simulink model "esercitazione3"  (R2023b)
settings: Solver=VariableStepAuto  StartTime=0.0  StopTime=12000  MaxStep=0.01  RelTol=1e-3
InitFcn:
  | init3
values from neighbouring files (symbols this model uses):
  B = 1.02e-9/60    (= 1.7e-11)    [init3.m]
  cp = 2*eps*sqrt(kp*mp)    [init3.m]
  d_sp = [0.001; 0.003; 0.005]    [init3.m]
  I = [I_x; I_y; I_z]    [init3.m]
  i = 0    [init3.m]
  Iw = Hm/wmax    (= 2.02922552442e-06)    [init3.m]
  Km = 1.09e-3    (= 0.00109)    [init3.m]
  kp = kt/(Lp^2)    (= 0.05)    [init3.m]
  Kprp = Km*Kv/Iw*20    (= 11.7098862172)    [init3.m]
  Kv = Km    (= 0.00109)    [init3.m]
  Lp = 0.2    [init3.m]
  mp = 0.146    [init3.m]
  mu = 398600    [init3.m]
  q_0 = [1; 0; 0; 0]    [init3.m]
  r_o = h+R_E    (= 7095.14)    [init3.m]
  Rm = 8.8    [init3.m]
  w_ic = [0; -w_o; 0]    [init3.m]
  w_o = sqrt(mu/(h+R_E)^3)    [init3.m]
  y_0 = [0; -w_o; 0; 0; 0]    [init3.m]
undefined symbols (not defined in the file or in its folder): C_phi, C_psi, C_theta
libraries: simulink x4, matrix_library x1
settings Model: Creator=dario  LastModifiedBy=Francesco

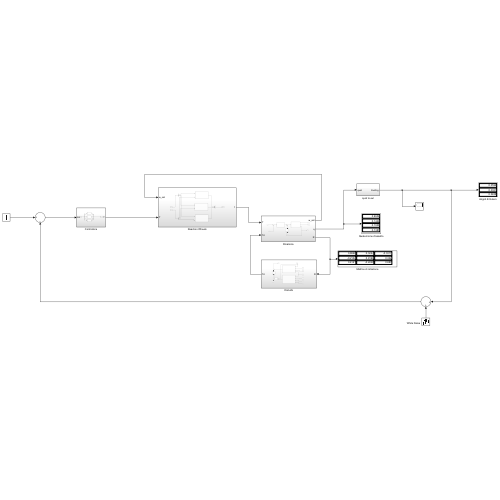
[thumbnail: Simulink's stored preview of the top-level diagram]
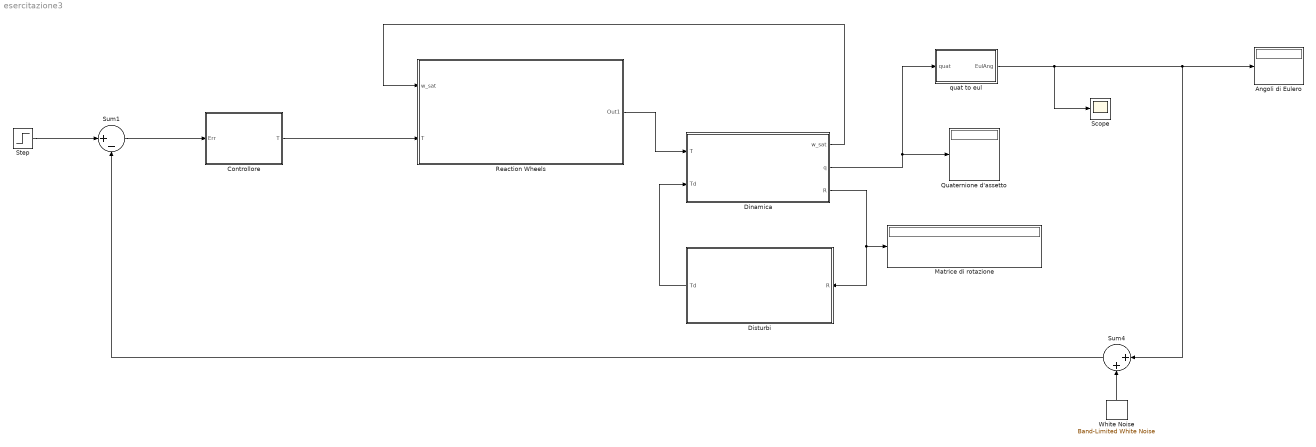
== system esercitazione3 ==
  " White Noise" : simulink/Sources/Band-Limited White Noise  Cov=[1e-6]  Ts=0.1  seed=[23341]
  Angoli di Eulero : Display
  Controllore : Subsystem
  Dinamica : Subsystem
  Disturbi : Subsystem
  Matrice di rotazione : Display
  Quaternione d'assetto : Display
  Reaction Wheels : Subsystem
  Scope : Scope
  Step : Step  After=20*pi/180  SampleTime=0  VectorParams1D=off
  Sum1 : Sum  Inputs=|+-
  Sum4 : Sum  Inputs=|++
  quat to eul : Subsystem
  wires:
  quat to eul/1(EulAng) -> Sum4/1, Angoli di Eulero/1, Scope/1
  Step/1 -> Sum1/1
  Sum1/1 -> Controllore/1(Err)
  Dinamica/2(q) -> quat to eul/1(quat), Quaternione d'assetto/1
  Controllore/1(T) -> Reaction Wheels/2(T)
  Dinamica/3(R) -> Disturbi/1(R), Matrice di rotazione/1
  Disturbi/1(Td) -> Dinamica/2(Td)
  " White Noise"/1 -> Sum4/2
  Sum4/1 -> Sum1/2
  Reaction Wheels/1(Out1) -> Dinamica/1(T)
  Dinamica/1(w_sat) -> Reaction Wheels/1(w_sat)

== system esercitazione3/Controllore ==
  Err : Inport
  C_phi : ZeroPole  Zeros=-0.00107058950149057  Poles=-1.61866208436204  Gain=C_phi.K
  C_psi : ZeroPole  Zeros=-0.000407767798417688  Poles=-1.39195940880825  Gain=C_psi.K
  C_th : ZeroPole  Zeros=-0.000686475078764194  Poles=-0.555984695028282  Gain=C_theta.K
  Demux : Demux  Outputs=3
  Mux : Mux  Inputs=3
  T : Outport
  wires:
  Demux/1 -> C_phi/1
  C_th/1 -> Mux/2
  C_psi/1 -> Mux/3
  Demux/3 -> C_psi/1
  Err/1 -> Demux/1
  Demux/2 -> C_th/1
  C_phi/1 -> Mux/1
  Mux/1 -> T/1

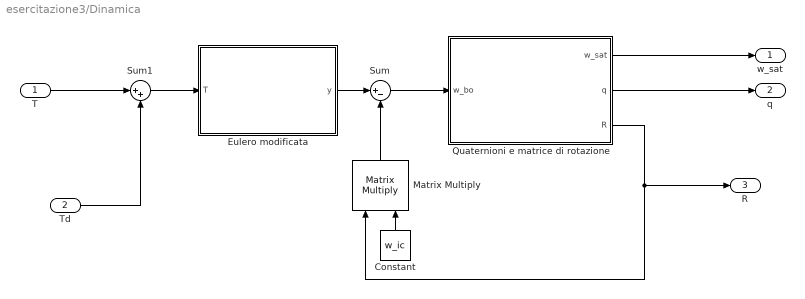
== system esercitazione3/Dinamica ==
  T : Inport
  Td : Inport  Port=2
  Constant : Constant  Value=w_ic  VectorParams1D=off
  "Eulero modificata " : Subsystem
  Matrix Multiply : Product  Inputs=**  Multiplication=Matrix(*)
  Quaternioni e matrice di rotazione : Subsystem
  Sum : Sum  Inputs=|+-
  Sum1 : Sum  Inputs=|++
  w_sat : Outport
  q : Outport  Port=2
  R : Outport  Port=3
  wires:
  Sum/1 -> Quaternioni e matrice di rotazione/1(w_bo)
  Constant/1 -> Matrix Multiply/2
  Quaternioni e matrice di rotazione/2(q) -> q/1
  Quaternioni e matrice di rotazione/3(R) -> R/1, Matrix Multiply/1
  Matrix Multiply/1 -> Sum/2
  T/1 -> Sum1/1
  Td/1 -> Sum1/2
  Sum1/1 -> "Eulero modificata "/1(T)
  "Eulero modificata "/1(y) -> Sum/1
  Quaternioni e matrice di rotazione/1(w_sat) -> w_sat/1

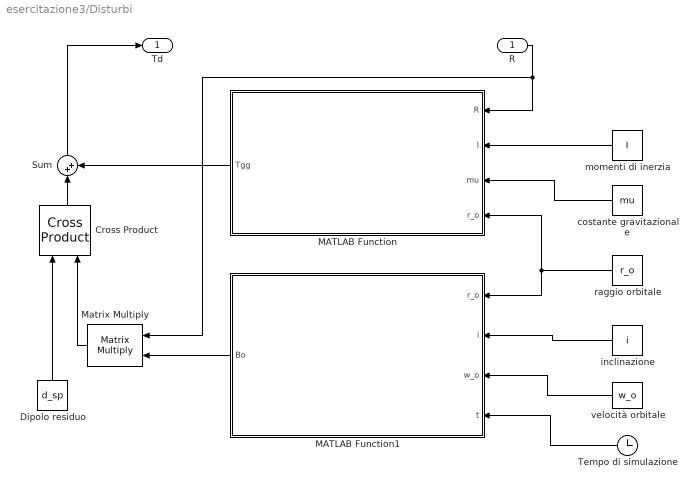
== system esercitazione3/Disturbi ==
  R : Inport
  Cross Product : matrix_library/Cross Product
  Dipolo residuo : Constant  Value=d_sp  VectorParams1D=off
  MATLAB Function : MATLAB Function  TreatAsAtomicUnit=on
  MATLAB Function1 : MATLAB Function  TreatAsAtomicUnit=on
  Matrix Multiply : Product  Inputs=**  Multiplication=Matrix(*)
  Sum : Sum  Inputs=|++
  Tempo di simulazione : Clock
  costante gravitazionale : Constant  Value=mu  VectorParams1D=off
  inclinazione : Constant  Value=i  VectorParams1D=off
  momenti di inerzia : Constant  Value=I  VectorParams1D=off
  raggio orbitale : Constant  Value=r_o  VectorParams1D=off
  velocità orbitale : Constant  Value=w_o  VectorParams1D=off
  Td : Outport
  wires:
  Tempo di simulazione/1 -> MATLAB Function1/4(t)
  raggio orbitale/1 -> MATLAB Function/4(r_o), MATLAB Function1/1(r_o)
  costante gravitazionale/1 -> MATLAB Function/3(mu)
  momenti di inerzia/1 -> MATLAB Function/2(I)
  MATLAB Function/1(Tgg) -> Sum/2
  R/1 -> MATLAB Function/1(R), Matrix Multiply/1
  velocità orbitale/1 -> MATLAB Function1/3(w_o)
  Dipolo residuo/1 -> Cross Product/1
  inclinazione/1 -> MATLAB Function1/2(i)
  Cross Product/1 -> Sum/1
  MATLAB Function1/1(Bo) -> Matrix Multiply/2
  Matrix Multiply/1 -> Cross Product/2
  Sum/1 -> Td/1

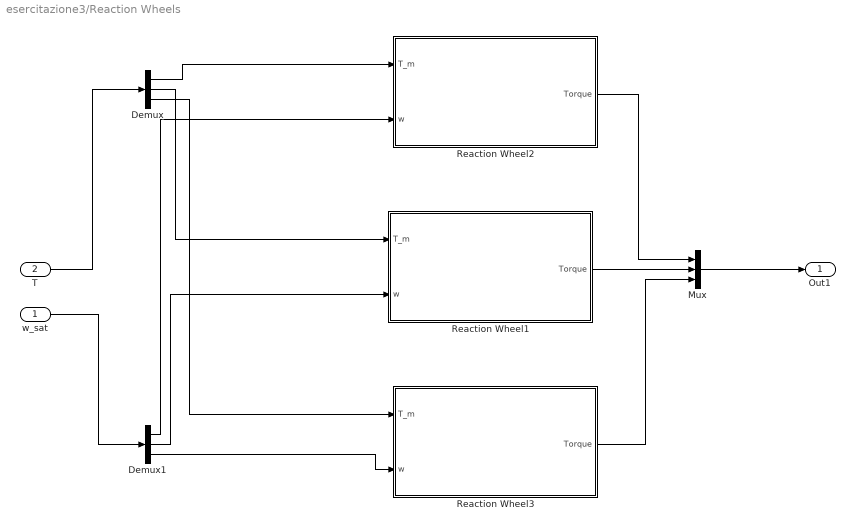
== system esercitazione3/Reaction Wheels ==
  w_sat : Inport
  T : Inport  Port=2
  Demux : Demux  Outputs=3
  Demux1 : Demux  Outputs=3
  Mux : Mux  Inputs=3
  Reaction Wheel1 : Subsystem
  Reaction Wheel2 : Subsystem
  Reaction Wheel3 : Subsystem
  Out1 : Outport
  wires:
  Demux/2 -> Reaction Wheel1/1(T_m)
  Reaction Wheel1/1(Torque) -> Mux/2
  Reaction Wheel2/1(Torque) -> Mux/1
  Demux1/3 -> Reaction Wheel3/2(w)
  Demux1/1 -> Reaction Wheel2/2(w)
  Demux1/2 -> Reaction Wheel1/2(w)
  T/1 -> Demux/1
  Mux/1 -> Out1/1
  Demux/1 -> Reaction Wheel2/1(T_m)
  Demux/3 -> Reaction Wheel3/1(T_m)
  w_sat/1 -> Demux1/1
  Reaction Wheel3/1(Torque) -> Mux/3

== system esercitazione3/quat to eul ==
  quat : Inport
  Attitude Matrix (Quaternion)1 : Subsystem
  Attitude Matrix to Euler Angles2 : Subsystem
  Demux : Demux
  Mux : Mux
  EulAng : Outport  VectorParamsAs1DForOutWhenUnconnected=off
  wires:
  Attitude Matrix to Euler Angles2/1(EulAng) -> EulAng/1
  Attitude Matrix (Quaternion)1/1(R_ob) -> Attitude Matrix to Euler Angles2/1(R_rb)
  quat/1 -> Demux/1
  Mux/1 -> Attitude Matrix (Quaternion)1/1(quat)
  Demux/1 -> Mux/4
  Demux/2 -> Mux/1
  Demux/3 -> Mux/2
  Demux/4 -> Mux/3

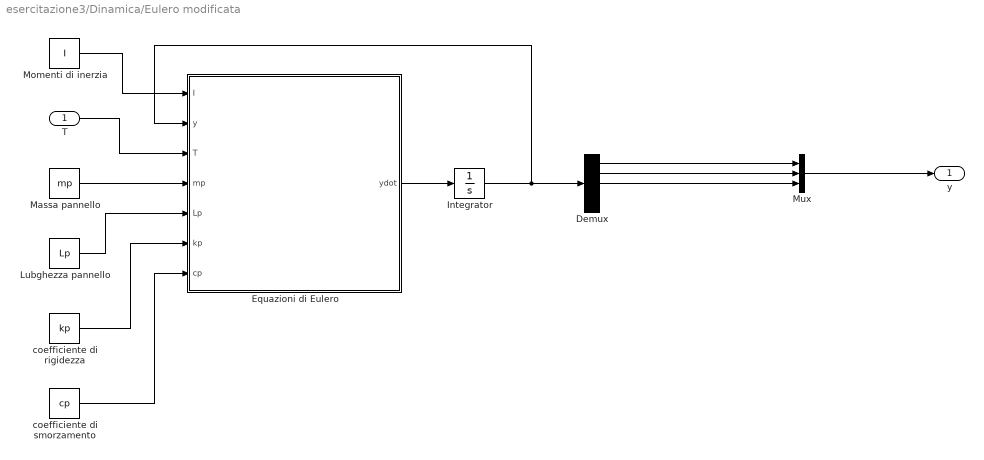
== system esercitazione3/Dinamica/Eulero modificata  ==
  T : Inport
  Demux : Demux  Outputs=5
  Equazioni di Eulero : MATLAB Function  TreatAsAtomicUnit=on
  Integrator : Integrator  InitialCondition=y_0
  Lubghezza pannello : Constant  Value=Lp  VectorParams1D=off
  Massa pannello : Constant  Value=mp  VectorParams1D=off
  Momenti di inerzia : Constant  Value=I  VectorParams1D=off
  Mux : Mux  Inputs=3
  coefficiente di rigidezza : Constant  Value=kp  VectorParams1D=off
  coefficiente di smorzamento : Constant  Value=cp  VectorParams1D=off
  y : Outport
  wires:
  Momenti di inerzia/1 -> Equazioni di Eulero/1(I)
  Equazioni di Eulero/1(ydot) -> Integrator/1
  T/1 -> Equazioni di Eulero/3(T)
  Massa pannello/1 -> Equazioni di Eulero/4(mp)
  Lubghezza pannello/1 -> Equazioni di Eulero/5(Lp)
  coefficiente di rigidezza/1 -> Equazioni di Eulero/6(kp)
  coefficiente di smorzamento/1 -> Equazioni di Eulero/7(cp)
  Demux/2 -> Mux/2
  Demux/1 -> Mux/1
  Demux/3 -> Mux/3
  Mux/1 -> y/1
  Integrator/1 -> Equazioni di Eulero/2(y), Demux/1

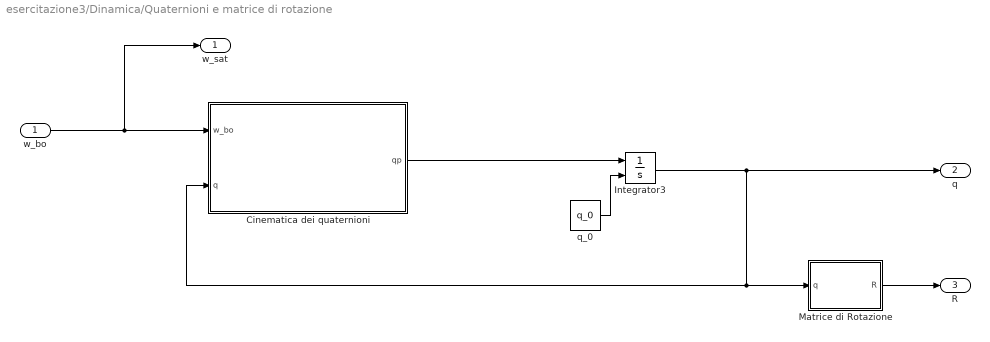
== system esercitazione3/Dinamica/Quaternioni e matrice di rotazione ==
  w_bo : Inport
  Cinematica dei quaternioni : MATLAB Function  TreatAsAtomicUnit=on
  Integrator3 : Integrator  InitialConditionSource=external
  Matrice di Rotazione : MATLAB Function  TreatAsAtomicUnit=on
  q_0 : Constant  Value=q_0  VectorParams1D=off
  w_sat : Outport
  q : Outport  Port=2
  R : Outport  Port=3
  wires:
  Integrator3/1 -> q/1, Cinematica dei quaternioni/2(q), Matrice di Rotazione/1(q)
  q_0/1 -> Integrator3/2
  Matrice di Rotazione/1(R) -> R/1
  Cinematica dei quaternioni/1(qp) -> Integrator3/1
  w_bo/1 -> w_sat/1, Cinematica dei quaternioni/1(w_bo)

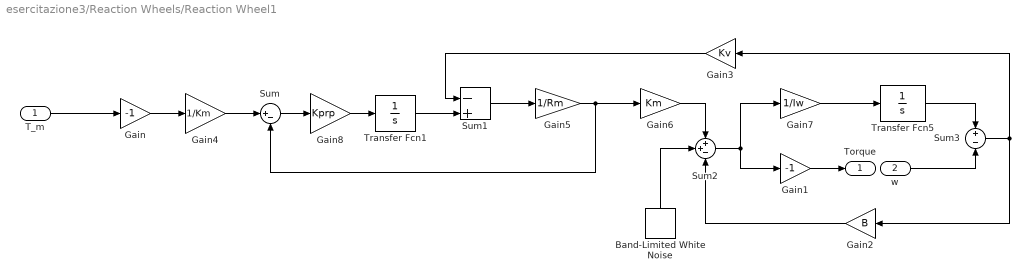
== system esercitazione3/Reaction Wheels/Reaction Wheel1 ==
  T_m : Inport
  w : Inport  Port=2
  Band-Limited White Noise : simulink/Sources/Band-Limited White Noise  Cov=[1e-13]  Ts=0.1  seed=[23341]
  Gain : Gain  Gain=-1
  Gain1 : Gain  Gain=-1
  Gain2 : Gain  Gain=B
  Gain3 : Gain  Gain=Kv
  Gain4 : Gain  Gain=1/Km
  Gain5 : Gain  Gain=1/Rm
  Gain6 : Gain  Gain=Km
  Gain7 : Gain  Gain=1/Iw
  Gain8 : Gain  Gain=Kprp
  Sum : Sum  Inputs=|+-
  Sum1 : Sum  Inputs=|-+
  Sum2 : Sum  Inputs=++-
  Sum3 : Sum  Inputs=+-
  Transfer Fcn1 : TransferFcn  Denominator=[1 0]
  Transfer Fcn5 : TransferFcn  Denominator=[1 0]
  Torque : Outport
  wires:
  Sum/1 -> Gain8/1
  Gain8/1 -> Transfer Fcn1/1
  Gain7/1 -> Transfer Fcn5/1
  Gain5/1 -> Gain6/1, Sum/2
  Gain4/1 -> Sum/1
  w/1 -> Sum3/2
  Gain1/1 -> Torque/1
  T_m/1 -> Gain/1
  Gain2/1 -> Sum2/3
  Transfer Fcn5/1 -> Sum3/1
  Gain3/1 -> Sum1/1
  Sum3/1 -> Gain3/1, Gain2/1
  Transfer Fcn1/1 -> Sum1/2
  Band-Limited White Noise/1 -> Sum2/2
  Gain/1 -> Gain4/1
  Sum1/1 -> Gain5/1
  Gain6/1 -> Sum2/1
  Sum2/1 -> Gain1/1, Gain7/1

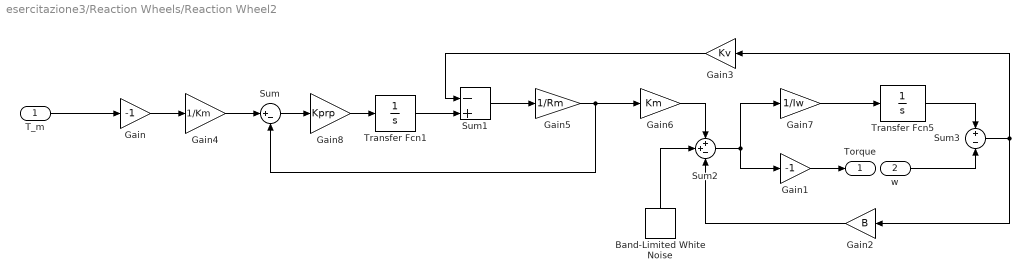
== system esercitazione3/Reaction Wheels/Reaction Wheel2 ==
  T_m : Inport
  w : Inport  Port=2
  Band-Limited White Noise : simulink/Sources/Band-Limited White Noise  Cov=[1e-13]  Ts=0.1  seed=[23341]
  Gain : Gain  Gain=-1
  Gain1 : Gain  Gain=-1
  Gain2 : Gain  Gain=B
  Gain3 : Gain  Gain=Kv
  Gain4 : Gain  Gain=1/Km
  Gain5 : Gain  Gain=1/Rm
  Gain6 : Gain  Gain=Km
  Gain7 : Gain  Gain=1/Iw
  Gain8 : Gain  Gain=Kprp
  Sum : Sum  Inputs=|+-
  Sum1 : Sum  Inputs=|-+
  Sum2 : Sum  Inputs=++-
  Sum3 : Sum  Inputs=+-
  Transfer Fcn1 : TransferFcn  Denominator=[1 0]
  Transfer Fcn5 : TransferFcn  Denominator=[1 0]
  Torque : Outport
  wires:
  Sum2/1 -> Gain7/1, Gain1/1
  Gain6/1 -> Sum2/1
  Sum1/1 -> Gain5/1
  Gain/1 -> Gain4/1
  Band-Limited White Noise/1 -> Sum2/2
  Transfer Fcn1/1 -> Sum1/2
  Sum3/1 -> Gain2/1, Gain3/1
  Gain3/1 -> Sum1/1
  Transfer Fcn5/1 -> Sum3/1
  Gain2/1 -> Sum2/3
  T_m/1 -> Gain/1
  Gain1/1 -> Torque/1
  w/1 -> Sum3/2
  Gain4/1 -> Sum/1
  Gain5/1 -> Sum/2, Gain6/1
  Gain7/1 -> Transfer Fcn5/1
  Gain8/1 -> Transfer Fcn1/1
  Sum/1 -> Gain8/1

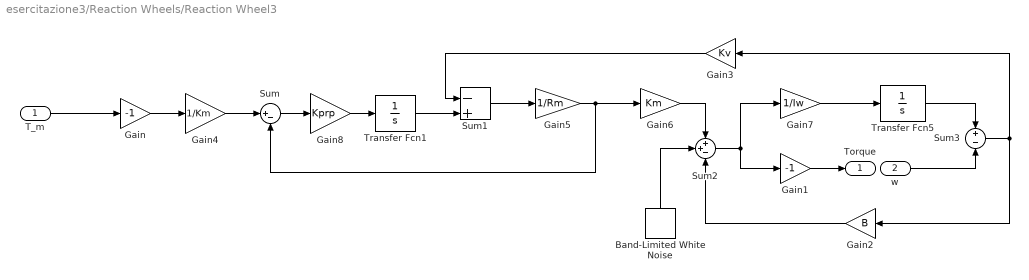
== system esercitazione3/Reaction Wheels/Reaction Wheel3 ==
  T_m : Inport
  w : Inport  Port=2
  Band-Limited White Noise : simulink/Sources/Band-Limited White Noise  Cov=[1e-13]  Ts=0.1  seed=[23341]
  Gain : Gain  Gain=-1
  Gain1 : Gain  Gain=-1
  Gain2 : Gain  Gain=B
  Gain3 : Gain  Gain=Kv
  Gain4 : Gain  Gain=1/Km
  Gain5 : Gain  Gain=1/Rm
  Gain6 : Gain  Gain=Km
  Gain7 : Gain  Gain=1/Iw
  Gain8 : Gain  Gain=Kprp
  Sum : Sum  Inputs=|+-
  Sum1 : Sum  Inputs=|-+
  Sum2 : Sum  Inputs=++-
  Sum3 : Sum  Inputs=+-
  Transfer Fcn1 : TransferFcn  Denominator=[1 0]
  Transfer Fcn5 : TransferFcn  Denominator=[1 0]
  Torque : Outport
  wires:
  Sum2/1 -> Gain7/1, Gain1/1
  Gain6/1 -> Sum2/1
  Sum1/1 -> Gain5/1
  Gain/1 -> Gain4/1
  Band-Limited White Noise/1 -> Sum2/2
  Transfer Fcn1/1 -> Sum1/2
  Sum3/1 -> Gain2/1, Gain3/1
  Gain3/1 -> Sum1/1
  Transfer Fcn5/1 -> Sum3/1
  Gain2/1 -> Sum2/3
  T_m/1 -> Gain/1
  Gain1/1 -> Torque/1
  w/1 -> Sum3/2
  Gain4/1 -> Sum/1
  Gain5/1 -> Sum/2, Gain6/1
  Gain7/1 -> Transfer Fcn5/1
  Gain8/1 -> Transfer Fcn1/1
  Sum/1 -> Gain8/1

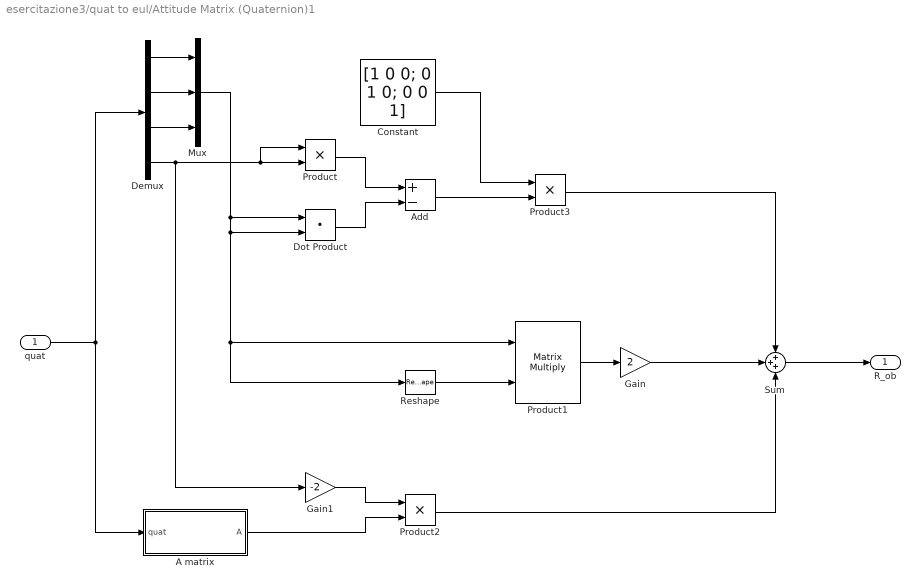
== system esercitazione3/quat to eul/Attitude Matrix (Quaternion)1 ==
  quat : Inport
  A matrix : Subsystem
  Add : Sum  Inputs=+-
  Constant : Constant  Value=[1 0 0; 0 1 0; 0 0 1]
  Demux : Demux
  Dot Product : DotProduct  OutDataTypeStr=Inherit: Inherit via internal rule
  Gain : Gain  Gain=2
  Gain1 : Gain  Gain=-2
  Mux : Mux  Inputs=3
  Product : Product  RndMeth=Zero
  Product1 : Product  Multiplication=Matrix(*)  RndMeth=Zero
  Product2 : Product  RndMeth=Zero
  Product3 : Product  RndMeth=Zero
  Reshape : Reshape  OutputDimensionality=Row vector (2-D)
  Sum : Sum  Inputs=+++
  R_ob : Outport  VectorParamsAs1DForOutWhenUnconnected=off
  wires:
  quat/1 -> Demux/1, A matrix/1(quat)
  Demux/4 -> Product/2, Product/1, Gain1/1
  Reshape/1 -> Product1/2
  Product1/1 -> Gain/1
  Gain/1 -> Sum/2
  Product/1 -> Add/1
  Dot Product/1 -> Add/2
  Product2/1 -> Sum/3
  Add/1 -> Product3/2
  Sum/1 -> R_ob/1
  Constant/1 -> Product3/1
  Product3/1 -> Sum/1
  Demux/1 -> Mux/1
  Demux/2 -> Mux/2
  Demux/3 -> Mux/3
  Mux/1 -> Dot Product/1, Reshape/1, Product1/1, Dot Product/2
  Gain1/1 -> Product2/1
  A matrix/1(A) -> Product2/2

== system esercitazione3/quat to eul/Attitude Matrix to Euler Angles2 ==
  R_rb : Inport
  Mux : Mux  Inputs=3
  Reshape : Reshape  OutputDimensionality=Column vector (2-D)
  cos(teta)>0 : Subsystem
  EulAng : Outport  VectorParamsAs1DForOutWhenUnconnected=off
  wires:
  cos(teta)>0/2(teta) -> Mux/2
  cos(teta)>0/1(phi) -> Mux/1
  cos(teta)>0/3(psi) -> Mux/3
  Mux/1 -> EulAng/1
  Reshape/1 -> cos(teta)>0/1(R_rb)
  R_rb/1 -> Reshape/1

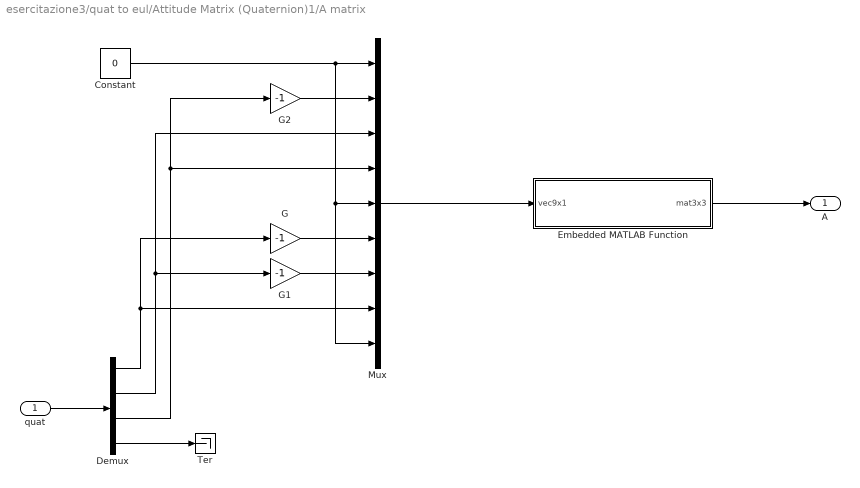
== system esercitazione3/quat to eul/Attitude Matrix (Quaternion)1/A matrix ==
  quat : Inport
  Constant : Constant  Value=0
  Demux : Demux
  Embedded MATLAB Function : MATLAB Function  TreatAsAtomicUnit=on
  G : Gain  Gain=-1
  G1 : Gain  Gain=-1
  G2 : Gain  Gain=-1
  Mux : Mux  Inputs=9
  Ter : Terminator
  A : Outport  VectorParamsAs1DForOutWhenUnconnected=off
  wires:
  Demux/4 -> Ter/1
  quat/1 -> Demux/1
  Constant/1 -> Mux/9, Mux/5, Mux/1
  Demux/1 -> G/1, Mux/8
  G1/1 -> Mux/7
  Demux/2 -> G1/1, Mux/3
  G/1 -> Mux/6
  G2/1 -> Mux/2
  Demux/3 -> G2/1, Mux/4
  Embedded MATLAB Function/1(mat3x3) -> A/1
  Mux/1 -> Embedded MATLAB Function/1(vec9x1)

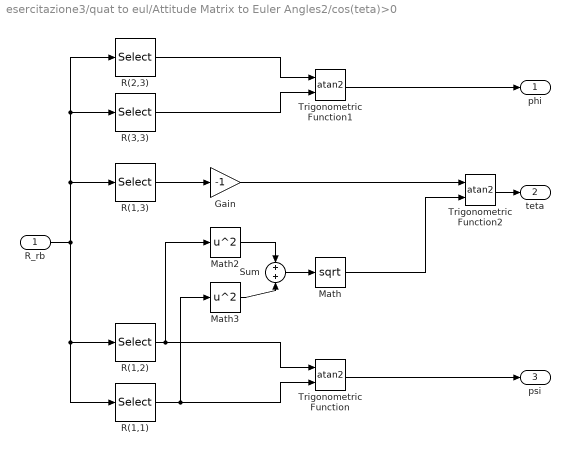
== system esercitazione3/quat to eul/Attitude Matrix to Euler Angles2/cos(teta)>0 ==
  R_rb : Inport
  Gain : Gain  Gain=-1
  Math : Math  Operator=sqrt  SignedPower=on
  Math2 : Math  Operator=square  SignedPower=on
  Math3 : Math  Operator=square  SignedPower=on
  R(1,1) : Selector  InputPortWidth=9  IndexOptions=Index vector (dialog)  Indices=[1]  OutputSizes=1
  R(1,2) : Selector  InputPortWidth=9  IndexOptions=Index vector (dialog)  Indices=[4]  OutputSizes=1
  R(1,3) : Selector  InputPortWidth=9  IndexOptions=Index vector (dialog)  Indices=[7]  OutputSizes=1
  R(2,3) : Selector  InputPortWidth=9  IndexOptions=Index vector (dialog)  Indices=[8]  OutputSizes=1
  R(3,3) : Selector  InputPortWidth=9  IndexOptions=Index vector (dialog)  Indices=[9]  OutputSizes=1
  Sum : Sum
  Trigonometric Function : Trigonometry  Operator=atan2
  Trigonometric Function1 : Trigonometry  Operator=atan2
  Trigonometric Function2 : Trigonometry  Operator=atan2
  phi : Outport  VectorParamsAs1DForOutWhenUnconnected=off
  teta : Outport  Port=2  VectorParamsAs1DForOutWhenUnconnected=off
  psi : Outport  Port=3  VectorParamsAs1DForOutWhenUnconnected=off
  wires:
  R_rb/1 -> R(1,1)/1, R(1,2)/1, R(1,3)/1, R(3,3)/1, R(2,3)/1
  R(1,2)/1 -> Trigonometric Function/1, Math2/1
  R(1,1)/1 -> Trigonometric Function/2, Math3/1
  R(2,3)/1 -> Trigonometric Function1/1
  R(3,3)/1 -> Trigonometric Function1/2
  R(1,3)/1 -> Gain/1
  Gain/1 -> Trigonometric Function2/1
  Math2/1 -> Sum/1
  Math3/1 -> Sum/2
  Sum/1 -> Math/1
  Math/1 -> Trigonometric Function2/2
  Trigonometric Function1/1 -> phi/1
  Trigonometric Function2/1 -> teta/1
  Trigonometric Function/1 -> psi/1

== matlab function esercitazione3/Dinamica/Quaternioni e matrice di rotazione/Cinematica dei quaternioni ==
  data: w_bo input; qp output; q input
function qp = Quaternioni(w_bo,q)
w_box=w_bo(1);
w_boy=w_bo(2);
w_boz=w_bo(3);

Q=[0 -w_box -w_boy -w_boz;
    w_box 0 w_boz -w_boy; 
    w_boy -w_boz 0 w_box; 
    w_boz w_boy -w_box 0];

qp=0.5*Q*q;

== matlab function esercitazione3/Dinamica/Eulero modificata /Equazioni di Eulero ==
  data: I input; y input; ydot output; T input; mp input; Lp input; kp input; cp input
function ydot = Eulero(I,y,T,mp,Lp,kp,cp)

%Equazioni di Eulero modificate per la presenza dei pannelli solari

wdotbix= -y(2)*y(3)*(I(3)-I(2))/(I(1)) + T(1)/I(1);

wdotbiy= -y(1)*y(3)*((I(1)-I(3))/I(2)) + T(2)/I(2);

wdotbiz= (y(1)*y(2)*(I(2)-I(1))-2*cp*Lp*y(4)-2*Lp*kp*y(5)-T(3))/(2*mp*Lp^2-I(3));

u2dot= (-mp*Lp*y(1)*y(2)*(I(2)-I(1))+I(3)*cp*y(4)+I(3)*kp*y(5)+T(3)*mp*Lp)/(2*mp^2*Lp^2-I(3)*mp);

udot= y(4);

ydot= [wdotbix; wdotbiy; wdotbiz; u2dot; udot];

== matlab function esercitazione3/Dinamica/Quaternioni e matrice di rotazione/Matrice di Rotazione ==
  data: q input; R output
function R = rotmat(q)
i=eye(3);
qdir=[q(2); q(3); q(4)];
A=[0 -q(4) q(3); q(4) 0 -q(2); -q(3) q(2) 0];
R=(q(1)^2-dot(qdir,qdir))*i+2*(qdir*qdir')-2*q(1)*A;

== matlab function esercitazione3/quat to eul/Attitude Matrix (Quaternion)1/A matrix/Embedded MATLAB Function ==
  data: vec9x1 input; mat3x3 output
function mat3x3 = vec2mat(vec9x1)
%#eml

s = size(vec9x1);

if s(1)>s(2)
    vec = vec9x1';
else
    vec = vec9x1;
end

mat3x3 = [vec(1:3); vec(4:6); vec(7:9)];

== matlab function esercitazione3/Disturbi/MATLAB Function ==
  data: R input; I input; Tgg output; mu input; r_o input
function Tgg = DisturboGrav(R, I, mu,r_o)

Tggx=(3*mu/r_o^3)*abs(I(3)-I(2))*R(2,3)*R(3,3);
Tggy=(-3*mu/r_o^3)*abs(I(3)-I(1))*R(1,3)*R(3,3);
Tggz=(-3*mu/r_o^3)*abs(I(1)-I(2))*R(1,3)*R(2,3);

Tgg = [Tggx; Tggy; Tggz];

== matlab function esercitazione3/Disturbi/MATLAB Function1 ==
  data: r_o input; Bo output; i input; w_o input; t input
function Bo = MagneticField(r_o,i,w_o,t)

B0 = 7.94e15/((r_o*1000)^3);

Box = B0*cos(i*sin(w_o*t))*sin(i*cos(w_o*t));
Boy = -B0*cos(i*sin(w_o*t))*cos(i*cos(w_o*t));
Boz = 2*B0*sin(i*sin(w_o*t));

Bo = [Box; Boy; Boz];
